simulink model "PRBS_doppio_sim"  (R2025b)
settings: Solver=ode45  StartTime=0.0  StopTime=20  RelTol=1e-3
undefined symbols (not defined in the file): DeltaT
libraries: slident x3
settings Model: Creator=USER  LastModifiedBy=francesco
settings SolverCC: AlgebraicLoopSolver=TrustRegion
settings DebuggingCC: UnconnectedInputMsg=warning  UnconnectedLineMsg=warning
settings ModelReferenceCC: EnableRefExpFcnMdlSchedulingChecks=on
settings RTWCC: GPUComputeCapability=3.5  DLArmComputeVersion=19.05

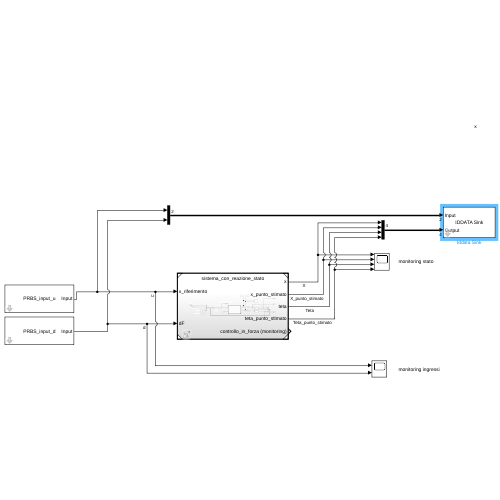
[thumbnail: Simulink's stored preview of the top-level diagram]
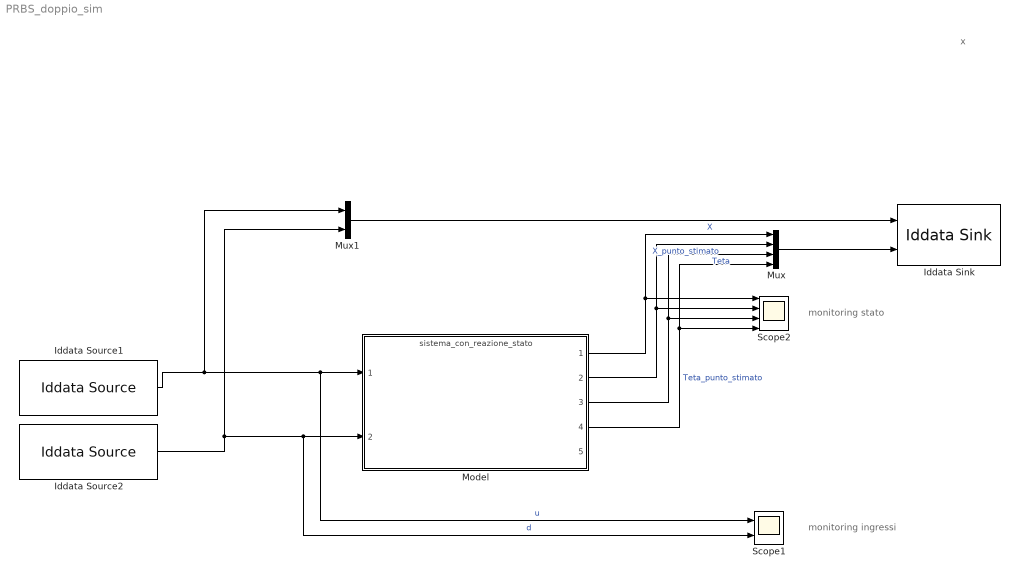
== system PRBS_doppio_sim ==
  note: monitoring stato
  note: monitoring ingressi
  note: x
  Iddata Sink : slident/Iddata Sink  datasetname=IO_ss  Ts=DeltaT  isu=on  isy=on
  Iddata Source1 : slident/Iddata Source  iddataobj=PRBS_input_u  T0=-1
  Iddata Source2 : slident/Iddata Source  iddataobj=PRBS_input_d  T0=-1
  Model : ModelReference  ModelNameDialog=sistema_con_reazione_stato.slx  SimulationMode=Normal  ModelReferenceVersion=9.56
  Mux : Mux
  Mux1 : Mux  Inputs=2
  Scope1 : Scope  NumInputPorts=2
      settings: ActiveDisplayYMinimum=-1.25  ActiveDisplayYMaximum=1.25
  Scope2 : Scope  NumInputPorts=4
      settings: ActiveDisplayYMinimum=-2.7821327849378408  ActiveDisplayYMaximum=2.7041990741135846  DataLoggingVariableName=ScopeData2
  wires:
  Model/1 -> Mux/1, Scope2/1  "X"
  Iddata Source2/1 -> Scope1/2, Model/2, Mux1/2  "d"
  Iddata Source1/1 -> Model/1, Scope1/1, Mux1/1  "u"
  Model/2 -> Mux/2, Scope2/2  "X_punto_stimato"
  Model/3 -> Mux/3, Scope2/3  "Teta"
  Model/4 -> Mux/4, Scope2/4  "Teta_punto_stimato"
  Mux/1 -> Iddata Sink/2
  Mux1/1 -> Iddata Sink/1
